simulink model "model1"  (R2024a)
settings: Solver=VariableStepAuto  StartTime=0.0  StopTime=10.0  RelTol=1e-3
values from neighbouring files (symbols this model uses):
  A = [8  1  11; 4  0  4 ; -4 -3  -7;]    [script1.m]
  B = [-1; -3; 3]    [script1.m]
  K = [0 K2] * P_real^-1    [script1.m]
settings Model: Creator=eva  LastModifiedBy=eva

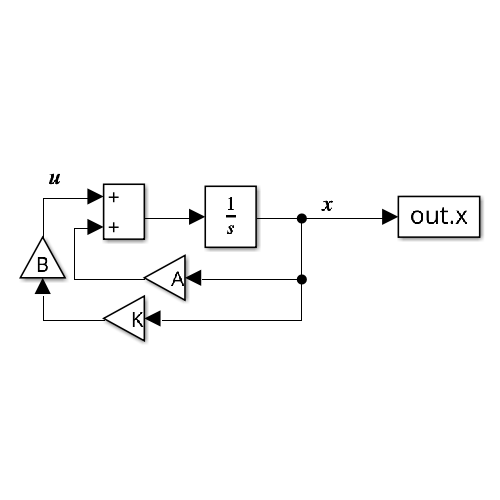
[thumbnail: Simulink's stored preview of the top-level diagram]
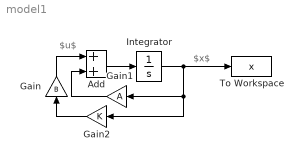
== system model1 ==
  note: $u$
  note: $x$
  Add : Sum
  Gain : Gain  Gain=B
  Gain1 : Gain  Gain=A
  Gain2 : Gain  Gain=K
  Integrator : Integrator
  To Workspace : ToWorkspace  VariableName=x  SaveFormat=Structure With Time  SampleTime=-1
  wires:
  Integrator/1 -> Gain2/1, Gain1/1, To Workspace/1
  Gain/1 -> Add/1
  Gain1/1 -> Add/2
  Add/1 -> Integrator/1
  Gain2/1 -> Gain/1
